simulink model "EmergencyBrake_Module"  (R2025a)
settings: Solver=VariableStepAuto
undefined symbols (not defined in the file): D_emergency_m
settings Model: Creator=Quang Huy  LastModifiedBy=ASUS

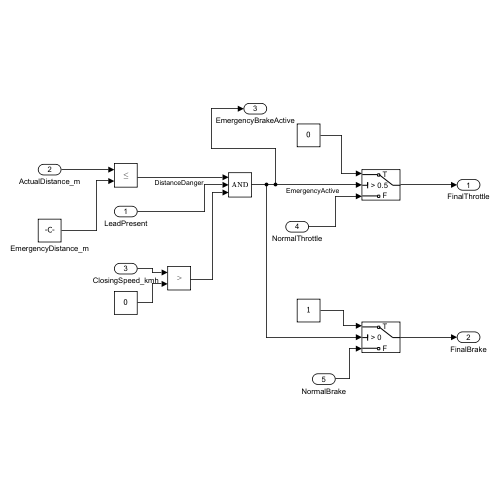
[thumbnail: Simulink's stored preview of the top-level diagram]
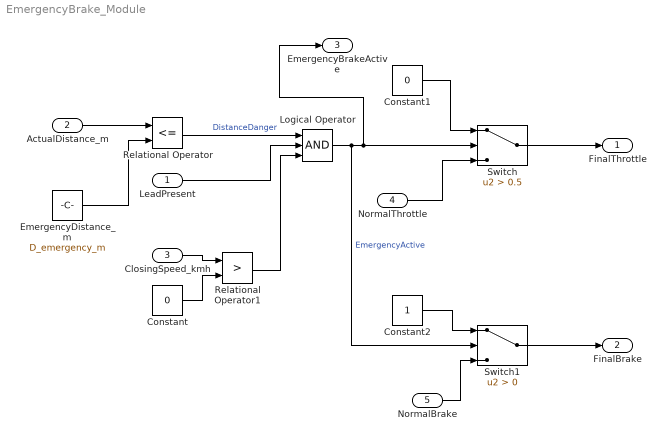
== system EmergencyBrake_Module ==
  LeadPresent : Inport
  ActualDistance_m : Inport  Port=2
  ClosingSpeed_kmh : Inport  Port=3
  NormalThrottle : Inport  Port=4
  NormalBrake : Inport  Port=5
  Constant : Constant  Value=0
  Constant1 : Constant  Value=0
  Constant2 : Constant
  EmergencyDistance_m : Constant  Value=D_emergency_m
  Logical Operator : Logic  Inputs=3  AllPortsSameDT=off  OutDataTypeStr=boolean
  Relational Operator : RelationalOperator  Operator=<=  OutDataTypeStr=boolean  RndMeth=Simplest  InputSameDT=off
  Relational Operator1 : RelationalOperator  Operator=>  OutDataTypeStr=boolean  RndMeth=Simplest  InputSameDT=off
  Switch : Switch  Criteria=u2 > Threshold  Threshold=0.5  SaturateOnIntegerOverflow=off  InputSameDT=off
  Switch1 : Switch  Criteria=u2 > Threshold  SaturateOnIntegerOverflow=off  InputSameDT=off
  FinalThrottle : Outport
  FinalBrake : Outport  Port=2
  EmergencyBrakeActive : Outport  Port=3
  wires:
  ActualDistance_m/1 -> Relational Operator/1
  EmergencyDistance_m/1 -> Relational Operator/2
  Relational Operator/1 -> Logical Operator/1  "DistanceDanger"
  LeadPresent/1 -> Logical Operator/2
  ClosingSpeed_kmh/1 -> Relational Operator1/1
  Constant/1 -> Relational Operator1/2
  Relational Operator1/1 -> Logical Operator/3
  Logical Operator/1 -> Switch1/2, EmergencyBrakeActive/1, Switch/2  "EmergencyActive"
  Constant1/1 -> Switch/1
  NormalThrottle/1 -> Switch/3
  Switch/1 -> FinalThrottle/1
  Constant2/1 -> Switch1/1
  NormalBrake/1 -> Switch1/3
  Switch1/1 -> FinalBrake/1
